simulink model "B210_display"  (R2019a)
settings: Solver=FixedStepDiscrete  StartTime=0.0  StopTime=inf  RelTol=1e-3
libraries: commsdrhw_v2 x1
Description:
  | Before running this model, you should set a variable of t to specify sample time.
settings Model: ModifiedComment=longt -- Tue Jul 23 14:21:16 2019 -- Version 1.3  OrderedModelArguments=off  Creator=longt  LastModifiedBy=longt
settings Model: ModifiedHistory=|
  | longt -- Fri Feb 15 22:22:24 2019 -- Version 1.2
  | Add description.
  | 
  | longt -- Fri Feb 15 10:03:04 2019 -- Version 1.1
settings DataIOCC: SaveOutput=off  SignalLogging=off  DSMLogging=off  SaveTime=off  ReturnWorkspaceOutputs=off
settings DebuggingCC: ArithmeticOperatorsInVariantConditions=warning

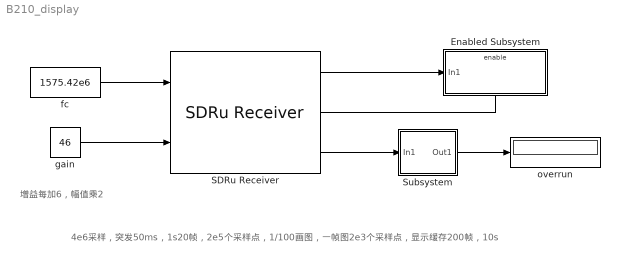
== system B210_display ==
  note: 增益每加6，幅值乘2
  note: 4e6采样，突发50ms，1s20帧，2e5个采样点，1/100画图，一帧图2e3个采样点，显示缓存200帧，10s
  Enabled Subsystem : Subsystem  TreatAsAtomicUnit=on
  SDRu Receiver : commsdrhw_v2/SDRu Receiver  rxtx=rx  initializeIPAddress=0  devMap=0  USRP2_IP=192.168.10.2  USRP_IP_X300=192.168.10.2  USRP_IP_X310=192.168.10.2  USRP_serialNumB200=No devices found  USRP_serialNumB210=315F337  platform=B210  prevPlatform=B210  lastIPAddressPopup=192.168.10.2  USRP_ID=315F337  LastIPAddress=192.168.10.2  ChannelMapping=1  centerFrequencySrc=Input port  centerFrequency=2.45e9  loOffsetSrc=Dialog  loOffset=0  gainSrc=Input port  gain=32  PPSSource=Internal  clockSource=Internal  masterClkRateParam=16000000  masterClkRateB200=32e6  masterClkRateB210=16e6  masterClkRateX300=200e6  masterClkRateX310=200e6  masterClkRate=100e6  decimInterpSrc=Dialog  decimInterp=4  USRP2_IP_NUM=[51 49 53 70 51 51 55]  TransportDataType=int16  overrunUnderrunPort=on  sampleTime=1/4e6  outputDatatype=Same as transport data type  frameLength=2e5  HOST_DATA_PORT=0  HOST_CONTROL_PORT=0  USRP2_DATA_PORT=0  USRP2_CONTROL_PORT=0  bufferMode=Continuous streaming  EnableBurstMode=on  NumFramesInBurst=1
      settings: SourceProductName=Communications Toolbox Support Package for USRP Radio  SourceProductBaseCode=USRP
  Subsystem : Subsystem
  fc : Constant  Value=1575.42e6  OutMin=70e6  OutMax=6000e6
  gain : Constant  Value=46  OutMin=-4  OutMax=71
  overrun : Display
  wires:
  fc/1 -> SDRu Receiver/1
  gain/1 -> SDRu Receiver/2
  SDRu Receiver/2 -> Enabled Subsystem/Enable
  SDRu Receiver/1 -> Enabled Subsystem/1(In1)
  Subsystem/1(Out1) -> overrun/1
  SDRu Receiver/3 -> Subsystem/1(In1)

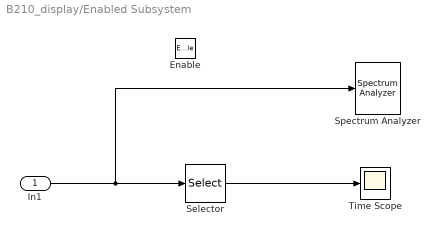
== system B210_display/Enabled Subsystem ==
  In1 : Inport
  Enable : EnablePort
  Selector : Selector  NumberOfDimensions=2  InputPortWidth=2  IndexOptions=Index vector (dialog),Index vector (dialog)  Indices=(1:2000)*100,1  OutputSizes=1,1
  Spectrum Analyzer : SpectrumAnalyzer
  Time Scope : Scope
  wires:
  In1/1 -> Spectrum Analyzer/1, Selector/1
  Selector/1 -> Time Scope/1

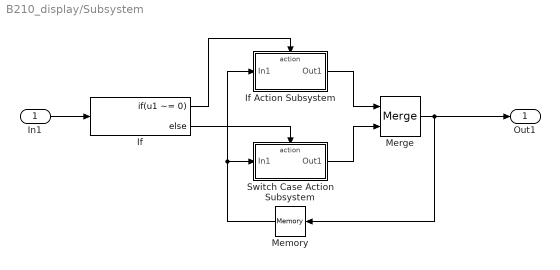
== system B210_display/Subsystem ==
  In1 : Inport
  If : If  IfExpression=u1 ~= 0
  If Action Subsystem : Subsystem  TreatAsAtomicUnit=on
  Memory : Memory
  Merge : Merge
  Switch Case Action Subsystem : Subsystem  TreatAsAtomicUnit=on
  Out1 : Outport
  wires:
  Switch Case Action Subsystem/1(Out1) -> Merge/2
  If Action Subsystem/1(Out1) -> Merge/1
  Merge/1 -> Out1/1, Memory/1
  Memory/1 -> Switch Case Action Subsystem/1(In1), If Action Subsystem/1(In1)
  In1/1 -> If/1
  If/1 -> If Action Subsystem/Action
  If/2 -> Switch Case Action Subsystem/Action

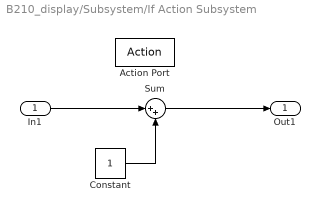
== system B210_display/Subsystem/If Action Subsystem ==
  In1 : Inport
  Action Port : ActionPort  ActionPortLabel=if(u1 ~= 0)
  Constant : Constant
  Sum : Sum  Inputs=|++
  Out1 : Outport
  wires:
  Sum/1 -> Out1/1
  In1/1 -> Sum/1
  Constant/1 -> Sum/2

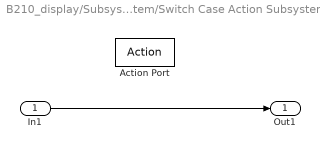
== system B210_display/Subsystem/Switch Case Action Subsystem ==
  In1 : Inport
  Action Port : ActionPort  ActionPortLabel=else
  Out1 : Outport
  wires:
  In1/1 -> Out1/1
